simulink model "simuladorsenoescalon"  (R2014a)
settings: Solver=ode45  StartTime=0.0  StopTime=10.0  RelTol=1e-3
settings Model: Creator=nigrobyte  LastModifiedBy=nigrobyte

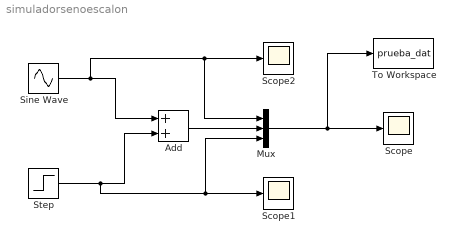
== system simuladorsenoescalon ==
  Add : Sum
  Mux : Mux  Inputs=3
  Scope : Scope
      settings: TimeRange=10  YMin=-1  YMax=2
  Scope1 : Scope
      settings: TimeRange=10  YMin=-1  YMax=2
  Scope2 : Scope
      settings: TimeRange=10  YMin=-1  YMax=2  SaveName=ScopeData2
  Sine Wave : Sin  SampleTime=0
  Step : Step  Time=5  SampleTime=0
  To Workspace : ToWorkspace  VariableName=prueba_dat  SampleTime=-1
  wires:
  Sine Wave/1 -> Mux/1, Scope2/1, Add/1
  Step/1 -> Mux/3, Scope1/1, Add/2
  Add/1 -> Mux/2
  Mux/1 -> To Workspace/1, Scope/1
